simulink model "Espacio_Estados_con_ROS_Trayectorias"  (R2021b)
settings: Solver=FixedStepAuto  StartTime=0.0  StopTime=t_final  FixedStep=T  RelTol=1e-3
undefined symbols (not defined in the file): A, B, C, D, Ke, Ki, Pose, T, Twist
libraries: robotlib x13, robotcorelib x1, simulink x1
settings Model: Creator=mluser  LastModifiedBy=esteven
settings SolverCC: AlgebraicLoopSolver=TrustRegion
settings DataIOCC: ReturnWorkspaceOutputs=off
settings DebuggingCC: SFMachineParentedDataDiag=warning

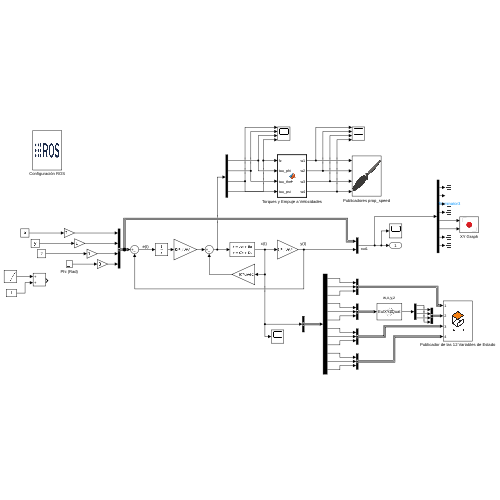
[thumbnail: Simulink's stored preview of the top-level diagram]
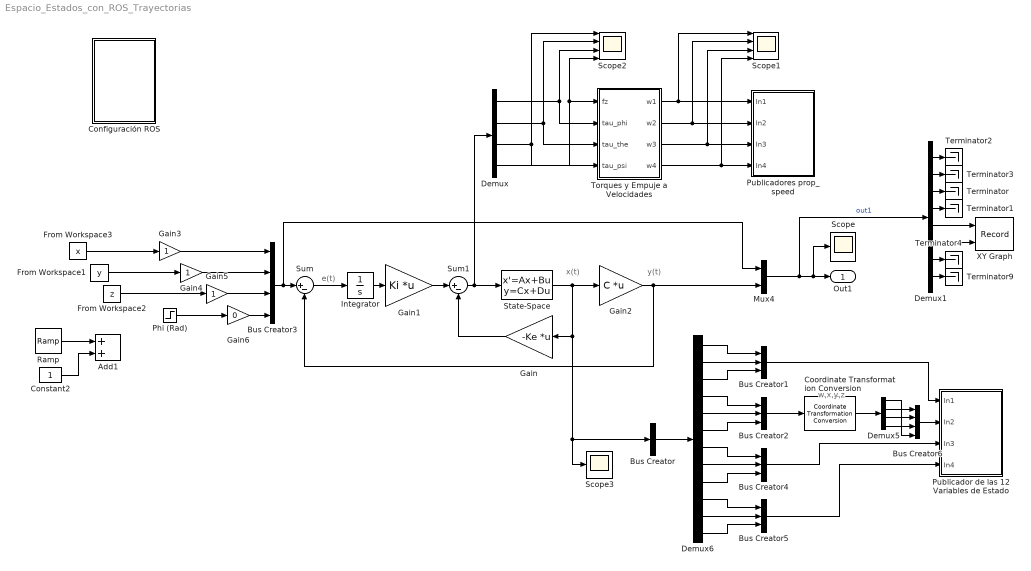
== system Espacio_Estados_con_ROS_Trayectorias ==
  note: e(t)
  note: y(t)
  note: x(t)
  note: w,x,y,z
  Add1 : Sum
  Bus Creator : BusCreator  Inputs=1
  Bus Creator{1..2,4..5} (4 alike) : BusCreator  Inputs=3
  Bus Creator3 : BusCreator  Inputs=4
  Bus Creator6 : BusCreator  Inputs=4
  Configuración ROS : Subsystem
      mask Display: image('$imagefile'); % Use "Edit Image" on toolstrip to change.
  Constant2 : Constant
  Coordinate Transformation Conversion : robotcorelib/Coordinate Transformation Conversion  InputRepresentation=Euler Angles  InputEulerSequence=XYZ  ShowTrVecInputPort=on  OutputRepresentation=Quaternion  OutputEulerSequence=ZYX  ShowTrVecOutputPort=on  SimulateUsing=Interpreted execution
      settings: SourceProductBaseCode=NV,RO,RR,UV
  Demux : Demux
  Demux1 : Demux  Outputs=8
  Demux5 : Demux
  Demux6 : Demux  Outputs=12
  From Workspace1 : FromWorkspace  VariableName=y  OutDataTypeStr=double  SampleTime=-1
  From Workspace2 : FromWorkspace  VariableName=z  OutDataTypeStr=double  SampleTime=-1
  From Workspace3 : FromWorkspace  VariableName=x  OutDataTypeStr=double  SampleTime=-1
  Gain : Gain  Gain=-Ke  Multiplication=Matrix(K*u) (u vector)
  Gain1 : Gain  Gain=Ki  Multiplication=Matrix(K*u) (u vector)
  Gain2 : Gain  Gain=C  Multiplication=Matrix(K*u) (u vector)
  Gain3 : Gain
  Gain4 : Gain
  Gain5 : Gain
  Gain6 : Gain  Gain=0
  Integrator : Integrator
  Mux4 : Mux  Inputs=2
  Phi (Rad) : Step  Time=3  SampleTime=T
  Publicador de las 12 Variables de Estado : Subsystem
      mask Display: image('$imagefile'); % Use "Edit Image" on toolstrip to change.
  Publicadores prop_speed : Subsystem
      mask Display: image('$imagefile'); % Use "Edit Image" on toolstrip to change.
  Ramp : simulink/Sources/Ramp  slope=0.25  start=5  InitialOutput=0
  Scope : Scope
  Scope1 : Scope  NumInputPorts=4
  Scope2 : Scope  NumInputPorts=4
  Scope3 : Scope
  State-Space : StateSpace  A=A  B=B  C=eye(12)  D=D  InitialCondition=0  ParameterTunability=Unconstrained
  Sum : Sum  Inputs=|+-
  Sum1 : Sum  Inputs=|+-
  Terminator{,1..4,9} (6 alike) : Terminator
  Torques y Empuje a Velocidades : MATLAB Function  TreatAsAtomicUnit=on
  XY Graph : Record  FileSettingsInternal="{\"entries\":[{\"content\":{\"excelSettings\":{\"content\":{},\"type\":\"Streamout.ExcelSettings\"}},\"type\":\"Streamout.FileSettingStorage\",\"uuid\":\"371dd3e1-4df5-4544-a34c-bee36d35162e\"}],\"packageUris\":[\"http://schema.mathworks.com/mf0/streamout_blocks/R2020a\"],\"version\":\"1.0\"}"  Layout=[1 1]  SignalsInternal="{\"entries\":[{\"content\":{\"signals\":[{\"content\":{\"blockPath\":[\"Espacio_Estados_con_ROS_Trayectorias/XY Graph\"],\"channel\":[],\"dimensions\":[1],\"domain\":\"Espacio_Estados_con_ROS_Trayectorias/XY Graph\",\"lineColor\":\"#a2142f\",\"plots\":[1],\"port\":1,\"sid\":[\"\"],\"signalID\":15780,\"signalName\":\"Demux1:5\"},\"type\":\"RecordBlkView.Signal\",\"uuid\":\"a5c647b6-96bc-40f4-8a37-98f45cc12f6f\"},{\"content\":{\"blockPath\":[\"Espacio_Estados_con_ROS_Trayectorias/XY Graph\"],\"channel\":[],\"dimensions\":[1],\"domain\":\"Espacio_Estados_con_ROS_Trayectorias/XY Graph\",\"lineColor\":\"#139fff\",\"plots\":[1],\"port\":2,\"sid\":[\"\"],\"signalID\":15784,\"signalName\":\"Demux1:6\"},\"type\":\"RecordBlkView.Signal\",\"uuid\":\"9432214f-6365-4998-b0a5-9ec0df72813b\"}]},\"type\":\"RecordBlkView.InputSignals\",\"uuid\":\"930269b1-3c4e-4ab2-b963-8e86b8c71482\"}],\"packageUris\":[\"http://schema.mathworks.com/mf0/streamout_blocks/R2020a\"],\"version\":\"1.0\"}"  VisualizationBindings="{\"xyplotplugin\":{\"info\":[{\"series\":[{\"bindingParametersList\":[{\"parameter\":\"X-Axis\",\"signalID\":15780,\"signalName\":\"Demux1:5\"},{\"parameter\":\"Y-Axis\",\"signalID\":15784,\"signalName\":\"Demux1:6\"}],\"seriesID\":16616}],\"subplotID\":1}]}}"  CompatibilityTag=XY
  Out1 : Outport
  wires:
  State-Space/1 -> Gain2/1, Scope3/1, Bus Creator/1, Gain/1
  Mux4/1 -> Demux1/1, Scope/1, Out1/1  "out1"
  Bus Creator3/1 -> Sum/1, Mux4/1
  Phi (Rad)/1 -> Gain6/1
  Sum/1 -> Integrator/1
  Sum1/1 -> Demux/1, State-Space/1
  Gain2/1 -> Mux4/2, Sum/2
  Gain/1 -> Sum1/2
  Integrator/1 -> Gain1/1
  Gain1/1 -> Sum1/1
  Torques y Empuje a Velocidades/1(w1) -> Publicadores prop_speed/1(In1), Scope1/1
  Torques y Empuje a Velocidades/2(w2) -> Publicadores prop_speed/2(In2), Scope1/2
  Torques y Empuje a Velocidades/3(w3) -> Publicadores prop_speed/3(In3), Scope1/3
  Torques y Empuje a Velocidades/4(w4) -> Publicadores prop_speed/4(In4), Scope1/4
  Demux/1 -> Scope2/3, Torques y Empuje a Velocidades/2(tau_phi)
  Demux/2 -> Scope2/2, Torques y Empuje a Velocidades/3(tau_the)
  Demux/3 -> Scope2/1, Torques y Empuje a Velocidades/4(tau_psi)
  Demux/4 -> Scope2/4, Torques y Empuje a Velocidades/1(fz)
  Bus Creator1/1 -> Publicador de las 12 Variables de Estado/1(In1)
  Demux6/1 -> Bus Creator1/1
  Demux6/2 -> Bus Creator1/2
  Demux6/3 -> Bus Creator1/3
  Demux6/4 -> Bus Creator2/1
  Demux6/5 -> Bus Creator2/2
  Demux6/6 -> Bus Creator2/3
  Bus Creator4/1 -> Publicador de las 12 Variables de Estado/3(In3)
  Demux6/7 -> Bus Creator4/1
  Demux6/8 -> Bus Creator4/2
  Demux6/9 -> Bus Creator4/3
  Demux6/10 -> Bus Creator5/1
  Demux6/11 -> Bus Creator5/2
  Demux6/12 -> Bus Creator5/3
  Bus Creator5/1 -> Publicador de las 12 Variables de Estado/4(In4)
  Demux5/2 -> Bus Creator6/1
  Bus Creator2/1 -> Coordinate Transformation Conversion/1
  Demux5/3 -> Bus Creator6/2
  Demux5/4 -> Bus Creator6/3
  Demux5/1 -> Bus Creator6/4
  Coordinate Transformation Conversion/1 -> Demux5/1
  Bus Creator6/1 -> Publicador de las 12 Variables de Estado/2(In2)
  Bus Creator/1 -> Demux6/1
  Gain3/1 -> Bus Creator3/1
  Gain4/1 -> Bus Creator3/2
  Gain5/1 -> Bus Creator3/3
  Gain6/1 -> Bus Creator3/4
  From Workspace3/1 -> Gain3/1
  From Workspace1/1 -> Gain4/1
  Constant2/1 -> Add1/2
  Ramp/1 -> Add1/1
  Demux1/3 -> Terminator/1
  Demux1/4 -> Terminator1/1
  Demux1/7 -> Terminator4/1
  Demux1/8 -> Terminator9/1
  Demux1/1 -> Terminator2/1
  Demux1/2 -> Terminator3/1
  Demux1/5 -> XY Graph/1
  Demux1/6 -> XY Graph/2
  From Workspace2/1 -> Gain5/1

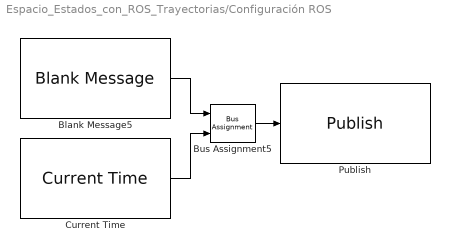
== system Espacio_Estados_con_ROS_Trayectorias/Configuración ROS ==
  Blank Message5 : robotlib/Blank Message  messageClass=Message  entityType=rosgraph_msgs/Clock  messageType=rosgraph_msgs/Clock  SampleTime=inf  legacyBusStruct=off
  Bus Assignment5 : BusAssignment  AssignedSignals=Clock_
  Current Time : robotlib/Current Time  OutputFormat=bus  SampleTime=-1  ModelName=Espacio_Estados_con_ROS_Trayectorias
      settings: SourceProductBaseCode=RR
  Publish : robotlib/Publish  topicSource=Select from ROS network  topic=/clock  messageType=rosgraph_msgs/Clock  legacyBusStruct=off  messageQueueLength=1
  wires:
  Blank Message5/1 -> Bus Assignment5/1
  Current Time/1 -> Bus Assignment5/2
  Bus Assignment5/1 -> Publish/1

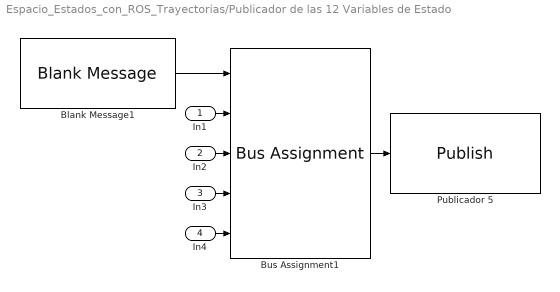
== system Espacio_Estados_con_ROS_Trayectorias/Publicador de las 12 Variables de Estado ==
  In1 : Inport
  In2 : Inport  Port=2
  In3 : Inport  Port=3
  In4 : Inport  Port=4
  Blank Message1 : robotlib/Blank Message  messageClass=Message  entityType=gazebo_msgs/ModelState  messageType=gazebo_msgs/ModelState  SampleTime=T  legacyBusStruct=off
  Bus Assignment1 : BusAssignment  AssignedSignals=Pose.Position,Pose.Orientation,Twist.Linear,Twist.Angular
  Publicador 5 : robotlib/Publish  topicSource=Specify your own  topic=/gazebo/model_state  messageType=gazebo_msgs/ModelState  legacyBusStruct=off  messageQueueLength=1
  wires:
  Bus Assignment1/1 -> Publicador 5/1
  In2/1 -> Bus Assignment1/3
  In4/1 -> Bus Assignment1/5
  Blank Message1/1 -> Bus Assignment1/1
  In3/1 -> Bus Assignment1/4
  In1/1 -> Bus Assignment1/2

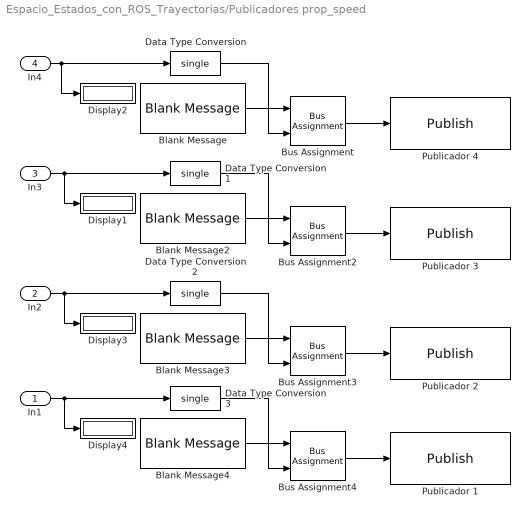
== system Espacio_Estados_con_ROS_Trayectorias/Publicadores prop_speed ==
  In1 : Inport
  In2 : Inport  Port=2
  In3 : Inport  Port=3
  In4 : Inport  Port=4
  Blank Message{,2..4} (4 alike) : robotlib/Blank Message  messageClass=Message  entityType=std_msgs/Float32  messageType=std_msgs/Float32  SampleTime=inf  legacyBusStruct=off
  Bus Assignment{,2..4} (4 alike) : BusAssignment  AssignedSignals=Data
  Data Type Conversion{,1..3} (4 alike) : DataTypeConversion  OutDataTypeStr=single
  Display{1..4} (4 alike) : Display
  Publicador 1 : robotlib/Publish  topicSource=Specify your own  topic=/qball/prop1_speed  messageType=std_msgs/Float32  legacyBusStruct=off  messageQueueLength=1
  Publicador 2 : robotlib/Publish  topicSource=Specify your own  topic=/qball/prop2_speed  messageType=std_msgs/Float32  legacyBusStruct=off  messageQueueLength=1
  Publicador 3 : robotlib/Publish  topicSource=Specify your own  topic=/qball/prop3_speed  messageType=std_msgs/Float32  legacyBusStruct=off  messageQueueLength=1
  Publicador 4 : robotlib/Publish  topicSource=Specify your own  topic=/qball/prop4_speed  messageType=std_msgs/Float32  legacyBusStruct=off  messageQueueLength=1
  wires:
  Data Type Conversion/1 -> Bus Assignment/2
  Blank Message3/1 -> Bus Assignment3/1
  Bus Assignment/1 -> Publicador 4/1
  In4/1 -> Display2/1, Data Type Conversion/1
  Bus Assignment3/1 -> Publicador 2/1
  Data Type Conversion2/1 -> Bus Assignment3/2
  Blank Message/1 -> Bus Assignment/1
  Data Type Conversion1/1 -> Bus Assignment2/2
  Blank Message2/1 -> Bus Assignment2/1
  Bus Assignment2/1 -> Publicador 3/1
  Data Type Conversion3/1 -> Bus Assignment4/2
  Blank Message4/1 -> Bus Assignment4/1
  Bus Assignment4/1 -> Publicador 1/1
  In2/1 -> Display3/1, Data Type Conversion2/1
  In3/1 -> Display1/1, Data Type Conversion1/1
  In1/1 -> Data Type Conversion3/1, Display4/1

== matlab function Espacio_Estados_con_ROS_Trayectorias/Torques y Empuje a Velocidades ==
  data: fz input; w1 output; tau_phi input; w2 output; w3 output; w4 output; tau_the input; tau_psi input
function [w1,w2,w3,w4] = H(fz,tau_phi,tau_the,tau_psi)
%         Salidas          Entradas

% Constantes 
l = 0.2;    % m
kf = 0.007; % Nm/A
km = 0.8;   % V/kRPM

% Matriz H
H = [kf     kf      kf      kf;
     0      l*kf    0       -l*kf;
     -l*kf  0       l*kf    0;  
     km     -km     km      -km];
 
% Inversa de H
H_inversa = inv(H);

% Vector de entrada
Torques = [fz;
           tau_phi;
           tau_the;
           tau_psi];
       
% Vector de salida      
Wi2 = H_inversa * Torques;


% Velocidades angulares al cuadrado
w1 = sqrt(abs(Wi2(1))) + 25;
w2 = sqrt(abs(Wi2(2))) + 25;
w3 = sqrt(abs(Wi2(3))) + 25;
w4 = sqrt(abs(Wi2(4))) + 25;


% Saturación de las velocidades angulares
RPM = 1020;
wmax = RPM*2*pi/60;
if w1>wmax
    w1 = wmax;
end
if w2>wmax
    w2 = wmax;
end
if w3>wmax
    w3 = wmax;
end
if w4>wmax
    w4 = wmax;
end
